simulink model "AM"  (R2021b)
settings: Solver=VariableStepAuto  StartTime=0.0  StopTime=5  MaxStep=0.00001  RelTol=1e-3
libraries: dsparch4 x1
settings Model: Creator=user  LastModifiedBy=user

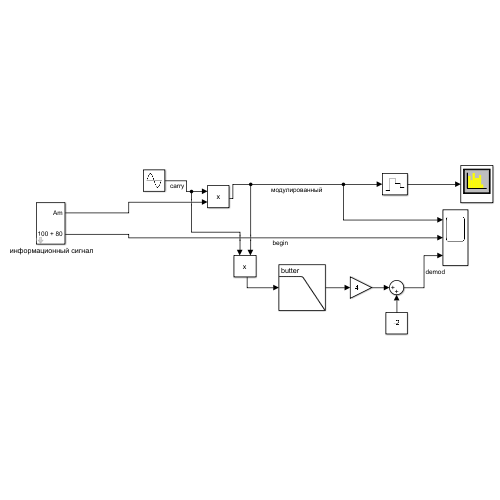
[thumbnail: Simulink's stored preview of the top-level diagram]
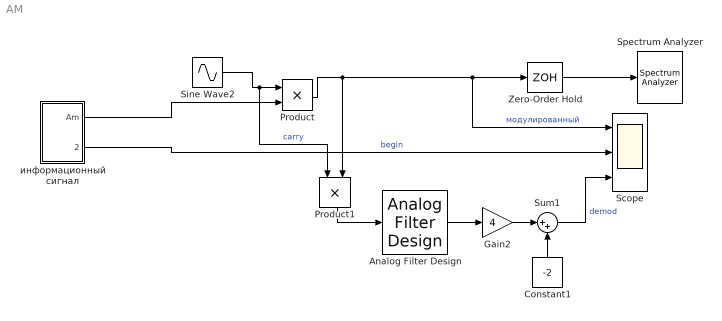
== system AM ==
  " информационный сигнал" : Subsystem  mask{m=0.5}
      mask prompts: m "modulation deep"
  Analog Filter Design : dsparch4/Analog Filter Design  method=Butterworth  filttype=Lowpass  N=8  Wlo=1000 * 2 * pi  Whi=80  Rp=2  Rs=40
  Constant1 : Constant  Value=-2
  Gain2 : Gain  Gain=4
  Product : Product
  Product1 : Product
  Scope : Scope  NumInputPorts=3
  Sine Wave2 : Sin  Frequency=1000 * 2 * pi  SampleTime=0
  Spectrum Analyzer : SpectrumAnalyzer
  Sum1 : Sum  Inputs=|++
  Zero-Order Hold : ZeroOrderHold  SampleTime=1/2500
  wires:
  Sine Wave2/1 -> Product1/1, Product/1  "carry"
  Product/1 -> Scope/1, Zero-Order Hold/1, Product1/2  "модулированный"
  Zero-Order Hold/1 -> Spectrum Analyzer/1
  Analog Filter Design/1 -> Gain2/1
  Gain2/1 -> Sum1/1
  Constant1/1 -> Sum1/2
  Product1/1 -> Analog Filter Design/1
  Sum1/1 -> Scope/3  "demod"
  " информационный сигнал"/1(Am) -> Product/2
  " информационный сигнал"/2(100 + 80) -> Scope/2  "begin"

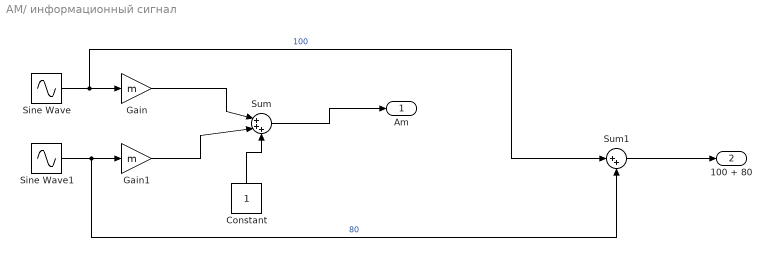
== system AM/ информационный сигнал ==
  Constant : Constant
  Gain : Gain  Gain=m
  Gain1 : Gain  Gain=m
  Sine Wave : Sin  Frequency=100 * 2* pi  SampleTime=0
  Sine Wave1 : Sin  Amplitude=1/4  Frequency=80*2*pi  SampleTime=0
  Sum : Sum  Inputs=|+++
  Sum1 : Sum  Inputs=|++
  Am : Outport
  100 + 80 : Outport  Port=2
  wires:
  Constant/1 -> Sum/3
  Gain1/1 -> Sum/2
  Sine Wave/1 -> Sum1/1, Gain/1  "100"
  Sine Wave1/1 -> Sum1/2, Gain1/1  "80"
  Gain/1 -> Sum/1
  Sum/1 -> Am/1
  Sum1/1 -> 100 + 80/1
